simulink model "vision_testing"  (R2013a)
settings: Solver=ode45  StartTime=0.0  StopTime=Inf  RelTol=1e-3
undefined symbols (not defined in the file or in its folder): none, Rec, SDTV, videoinput
libraries: visionsinks x7, visionconversions x1, imaqlib x1
settings Model: Creator=Michael  LastModifiedBy=Michael

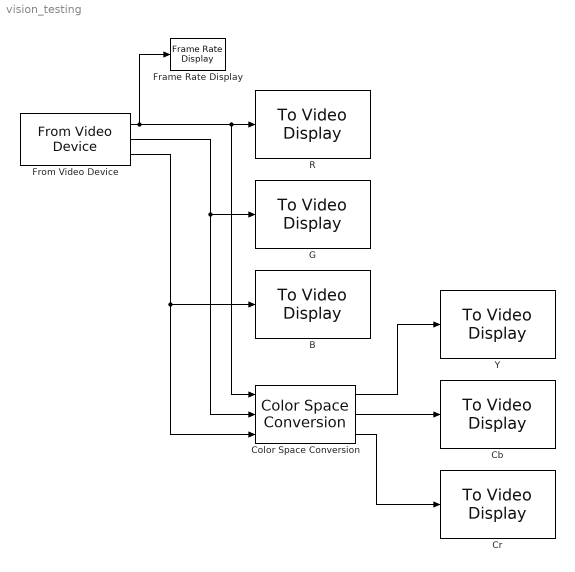
== system vision_testing ==
  B : visionsinks/To Video Display  inputType=Obsolete  imagePorts=One multidimensional signal  OutputDevice=On-screen video monitor  fullScreen=off  videoWindowX=682  videoWindowY=68  saveWindowSize=off  videoWindowWidth=640  videoWindowHeight=480  dataOrg=Column-major  openAtMdlStart=on  isWindowOpen=off  inputColorFormat=RGB
  Cb : visionsinks/To Video Display  inputType=Obsolete  imagePorts=One multidimensional signal  OutputDevice=On-screen video monitor  fullScreen=off  videoWindowX=44  videoWindowY=39  saveWindowSize=off  videoWindowWidth=44  videoWindowHeight=41  dataOrg=Column-major  openAtMdlStart=on  isWindowOpen=off  inputColorFormat=RGB
  Color Space Conversion : visionconversions/Color Space  Conversion  conversion=Obsolete  conversionActive=R'G'B' to Y'CbCr  wp_str=D65  rec=Rec. 601 (SDTV)  sys=1125/60/2:1  imagePorts=Separate color signals
  Cr : visionsinks/To Video Display  inputType=Obsolete  imagePorts=One multidimensional signal  OutputDevice=On-screen video monitor  fullScreen=off  videoWindowX=44  videoWindowY=39  saveWindowSize=off  videoWindowWidth=44  videoWindowHeight=41  dataOrg=Column-major  openAtMdlStart=on  isWindowOpen=off  inputColorFormat=RGB
  Frame Rate Display : visionsinks/Frame Rate Display  UpdateRate=10
  From Video Device : imaqlib/From Video Device  DeviceMenu=winvideo 1 (Lenovo EasyCamera)  Device=winvideo 1 (Lenovo EasyCamera)  ObjConstructor=videoinput('winvideo', 1)  VideoFormatMenu=YUY2_640x480  VideoFormat=YUY2_640x480  VideoSource=input1  ROIPosition=[0 0 480 640]  EnableHWTrigger=off  TriggerConfiguration=none/none  SampleTime=1/30  OutputPortsMode=Separate color signals  DataType=single  CanDoHWTrigger=no  ReturnedColorSpace=rgb  BlockHandle=604.0001  ROIWidth=640  ROIHeight=480  ROIColumn=0  ROIRow=0  EngXMLPath=C:\Program Files\MATLAB\R2013a\toolbox\imaq\imaq\private  DevXMLPath=C:\Program Files\MATLAB\R2013a\toolbox\imaq\imaqadaptors\win64  EngLibPath=C:\Program Files\MATLAB\R2013a\toolbox\imaq\imaqblks\imaqmex\win64  ColorSpace=rgb  BayerSensorAlignment=grbg
  G : visionsinks/To Video Display  inputType=Obsolete  imagePorts=One multidimensional signal  OutputDevice=On-screen video monitor  fullScreen=off  videoWindowX=89  videoWindowY=25  saveWindowSize=off  videoWindowWidth=640  videoWindowHeight=480  dataOrg=Column-major  openAtMdlStart=on  isWindowOpen=off  inputColorFormat=RGB
  R : visionsinks/To Video Display  inputType=Obsolete  imagePorts=One multidimensional signal  OutputDevice=On-screen video monitor  fullScreen=off  videoWindowX=382  videoWindowY=140  saveWindowSize=off  videoWindowWidth=640  videoWindowHeight=480  dataOrg=Column-major  openAtMdlStart=on  isWindowOpen=off  inputColorFormat=RGB
  Y : visionsinks/To Video Display  inputType=Obsolete  imagePorts=One multidimensional signal  OutputDevice=On-screen video monitor  fullScreen=off  videoWindowX=44  videoWindowY=39  saveWindowSize=off  videoWindowWidth=44  videoWindowHeight=41  dataOrg=Column-major  openAtMdlStart=on  isWindowOpen=off  inputColorFormat=RGB
  wires:
  From Video Device/1 -> Color Space Conversion/1, R/1, Frame Rate Display/1
  From Video Device/2 -> Color Space Conversion/2, G/1
  From Video Device/3 -> Color Space Conversion/3, B/1
  Color Space Conversion/1 -> Y/1
  Color Space Conversion/2 -> Cb/1
  Color Space Conversion/3 -> Cr/1
